simulink model "Demo_DSRC_DNPW_cs"  (Simulink 7.6)
settings: Solver=ode5  SolverMode=SingleTasking  StartTime=0.0  StopTime=5  FixedStep=1/20  RelTol=1e-3
PreLoadFcn:
  | check_NUTS_defined;
  | 
  | assignin('base',['model_closed_' bdroot],false);
InitFcn:
  | PreScanExperimentInitFcn(bdroot)
StopFcn:
  | PreScanExperimentStopFcn(bdroot)
undefined symbols (not defined in the file): DiscIntNeverNeededParam, spare_1, spare_10, spare_11, spare_12, spare_13, spare_14, spare_15, spare_16, spare_17, spare_18, spare_19, spare_2, spare_3, spare_4, spare_5, spare_6, spare_7, spare_8, spare_9
libraries: PreScanSimulinkLibrary x29, PreScanUsefulBlocks x11, simulink x9, simulink_extras x2
(part 5 of 6)

== system Demo_DSRC_DNPW_cs/STATE_Nissan_Cabstar_1/velRPY ==
  Y : Inport
  Assignment : Assignment  IndexMode=Zero-based  SampleTime=TimeStep  IndexOptions=Starting index (dialog)  Indices=PortIndex  OutputSizes=[1 1]
  Data Store Read : DataStoreRead  DataStoreName=SimCoreActuators  SampleTime=TimeStep
  Data Store Write : DataStoreWrite  DataStoreName=SimCoreActuators
  wires:
  Assignment/1 -> Data Store Write/1
  Data Store Read/1 -> Assignment/1
  Y/1 -> Assignment/2

== system Demo_DSRC_DNPW_cs/STATE_Toyota_Yaris_1/Acceleration ==
  Y : Inport
  Assignment : Assignment  IndexMode=Zero-based  SampleTime=TimeStep  IndexOptions=Starting index (dialog)  Indices=PortIndex  OutputSizes=[1 1]
  Data Store Read : DataStoreRead  DataStoreName=SimCoreActuators  SampleTime=TimeStep
  Data Store Write : DataStoreWrite  DataStoreName=SimCoreActuators
  wires:
  Assignment/1 -> Data Store Write/1
  Data Store Read/1 -> Assignment/1
  Y/1 -> Assignment/2

== system Demo_DSRC_DNPW_cs/STATE_Toyota_Yaris_1/Position ==
  Y : Inport
  Assignment : Assignment  IndexMode=Zero-based  SampleTime=TimeStep  IndexOptions=Starting index (dialog)  Indices=PortIndex  OutputSizes=[1 1]
  Data Store Read : DataStoreRead  DataStoreName=SimCoreActuators  SampleTime=TimeStep
  Data Store Write : DataStoreWrite  DataStoreName=SimCoreActuators
  wires:
  Y/1 -> Assignment/2
  Data Store Read/1 -> Assignment/1
  Assignment/1 -> Data Store Write/1

== system Demo_DSRC_DNPW_cs/STATE_Toyota_Yaris_1/RPY ==
  Y : Inport
  Assignment : Assignment  IndexMode=Zero-based  SampleTime=TimeStep  IndexOptions=Starting index (dialog)  Indices=PortIndex  OutputSizes=[1 1]
  Data Store Read : DataStoreRead  DataStoreName=SimCoreActuators  SampleTime=TimeStep
  Data Store Write : DataStoreWrite  DataStoreName=SimCoreActuators
  wires:
  Assignment/1 -> Data Store Write/1
  Data Store Read/1 -> Assignment/1
  Y/1 -> Assignment/2

== system Demo_DSRC_DNPW_cs/STATE_Toyota_Yaris_1/Velocity ==
  Y : Inport
  Assignment : Assignment  IndexMode=Zero-based  SampleTime=TimeStep  IndexOptions=Starting index (dialog)  Indices=PortIndex  OutputSizes=[1 1]
  Data Store Read : DataStoreRead  DataStoreName=SimCoreActuators  SampleTime=TimeStep
  Data Store Write : DataStoreWrite  DataStoreName=SimCoreActuators
  wires:
  Assignment/1 -> Data Store Write/1
  Data Store Read/1 -> Assignment/1
  Y/1 -> Assignment/2

== system Demo_DSRC_DNPW_cs/STATE_Toyota_Yaris_1/velRPY ==
  Y : Inport
  Assignment : Assignment  IndexMode=Zero-based  SampleTime=TimeStep  IndexOptions=Starting index (dialog)  Indices=PortIndex  OutputSizes=[1 1]
  Data Store Read : DataStoreRead  DataStoreName=SimCoreActuators  SampleTime=TimeStep
  Data Store Write : DataStoreWrite  DataStoreName=SimCoreActuators
  wires:
  Assignment/1 -> Data Store Write/1
  Data Store Read/1 -> Assignment/1
  Y/1 -> Assignment/2

== system Demo_DSRC_DNPW_cs/Toyota_Yaris_1/DSRC Transmitter ==
  Data : Inport
  Enable : EnablePort  PropagateVarSize=During execution
  DSRC_T_BusAssignment : BusAssignment  Tag=BusDSRCT  AssignedSignals=spare_1,spare_2,spare_3,spare_4,spare_5,spare_6,spare_7,spare_8,spare_9,spare_10,spare_11,spare_12,spare_13,spare_14,spare_15,spare_16,spare_17,spare_18,spare_19
  DSRC_T_Mux : Subsystem  Tag=MuxDSRCT
      settings: DeleteFcn=PreScanBlockDeleteFcn;
      mask Type: PreScan Mux Block:
      mask Display:
      | port_label('input', 1, 'Warning signal ID')
      | port_label('input', 2, 'Maneuvre ID')
      | port_label('input', 3, 'Vehicle Type')
      | port_label('input', 4, 'Braking Capacity')
      | port_label('input', 5, 'Vehicle Size')
      | port_label('input', 6, 'spare')
  Demux : Demux  Outputs=19
  Ground_{4..8} (5 alike) : Ground
  DSRC_T : Outport  Tag=AntennaTOutport
  wires:
  Demux/19 -> DSRC_T_BusAssignment/20  "Vehicle Height"
  Demux/18 -> DSRC_T_BusAssignment/19  "Vehicle Width"
  Demux/17 -> DSRC_T_BusAssignment/18  "Brakes"
  Demux/16 -> DSRC_T_BusAssignment/17  "Yaw rate"
  Demux/15 -> DSRC_T_BusAssignment/16  "Veritical Acc"
  Demux/14 -> DSRC_T_BusAssignment/15  "Lateral Acc"
  Demux/13 -> DSRC_T_BusAssignment/14  "Longitudinal Acc"
  Demux/12 -> DSRC_T_BusAssignment/13  "Angle"
  Demux/11 -> DSRC_T_BusAssignment/12  "Heading"
  Demux/10 -> DSRC_T_BusAssignment/11  "Speed"
  Demux/9 -> DSRC_T_BusAssignment/10  "Transmission State"
  Demux/8 -> DSRC_T_BusAssignment/9  "Accuracy"
  Demux/7 -> DSRC_T_BusAssignment/8  "Elevation"
  Demux/6 -> DSRC_T_BusAssignment/7  "Longitudinal"
  Demux/5 -> DSRC_T_BusAssignment/6  "Lateral"
  Ground_8/1 -> DSRC_T_Mux/5(vehicle_size)  "l50"
  Ground_7/1 -> DSRC_T_Mux/4(brakingcapacity)  "l49"
  Ground_6/1 -> DSRC_T_Mux/3(vehicle_type)  "l48"
  Ground_5/1 -> DSRC_T_Mux/2(maneuvre_id)  "l47"
  Ground_4/1 -> DSRC_T_Mux/1(warning_signal_id)  "l46"
  DSRC_T_Mux/1(Out1) -> DSRC_T/1  "l60"
  DSRC_T_BusAssignment/1 -> DSRC_T_Mux/6(spare)  "l58"
  Demux/4 -> DSRC_T_BusAssignment/5  "SecMark"
  Demux/3 -> DSRC_T_BusAssignment/4  "TempId"
  Demux/2 -> DSRC_T_BusAssignment/3  "MsgCount"
  Demux/1 -> DSRC_T_BusAssignment/2  "MsgId"
  Data/1 -> Demux/1
  DSRC_T_Mux/2(Out2) -> DSRC_T_BusAssignment/1  "L29"

== system Demo_DSRC_DNPW_cs/Toyota_Yaris_1/J2735 Encoder Basic Safety Message ==
  Msg : Inport
  Enable : EnablePort  PropagateVarSize=During execution
  Constant : Constant
  Demux : Demux  Outputs=19
  Embedded MATLAB Function : Stateflow chart  TreatAsAtomicUnit=on
  f() : Outport  InitialOutput=[1]
  Data : Outport  Port=2
  wires:
  Embedded MATLAB Function/1(y) -> Data/1
  Demux/19 -> Embedded MATLAB Function/19(u19)
  Demux/18 -> Embedded MATLAB Function/18(u18)
  Demux/17 -> Embedded MATLAB Function/17(u17)
  Demux/16 -> Embedded MATLAB Function/16(u16)
  Demux/15 -> Embedded MATLAB Function/15(u15)
  Demux/14 -> Embedded MATLAB Function/14(u14)
  Demux/13 -> Embedded MATLAB Function/13(u13)
  Demux/12 -> Embedded MATLAB Function/12(u12)
  Demux/11 -> Embedded MATLAB Function/11(u11)
  Demux/10 -> Embedded MATLAB Function/10(u10)
  Demux/9 -> Embedded MATLAB Function/9(u9)
  Demux/8 -> Embedded MATLAB Function/8(u8)
  Demux/7 -> Embedded MATLAB Function/7(u7)
  Demux/6 -> Embedded MATLAB Function/6(u6)
  Demux/5 -> Embedded MATLAB Function/5(u5)
  Demux/4 -> Embedded MATLAB Function/4(u4)
  Demux/3 -> Embedded MATLAB Function/3(u3)
  Demux/2 -> Embedded MATLAB Function/2(u2)
  Demux/1 -> Embedded MATLAB Function/1(u1)
  Constant/1 -> f()/1  "Enabled"
  Msg/1 -> Demux/1

== system Demo_DSRC_DNPW_cs/Toyota_Yaris_1/SELF_Demux ==
  SELF : Inport
  Demux1 : Demux  Outputs=3
  Demux2 : Demux  Outputs=3
  Demux3 : Demux  Outputs=[3 3 1 1]
  Demux4 : Demux  Outputs=3
  Gain : Gain  Gain=180/pi
  Gain1 : Gain  Gain=180/pi
  Selector : Selector  InputPortWidth=3  IndexOptions=Index vector (dialog)  Indices=[3]  OutputSizes=1
  compas converter : Subsystem
  xyz2GPS : PreScanUsefulBlocks/xyz2GPS  CoordinateCount=1  GPS_base=[0.000000 0.000000 0.000]
  x [m] : Outport
  y [m] : Outport  Port=2
  z [m] : Outport  Port=3
  rotx [deg] : Outport  Port=4
  roty [deg] : Outport  Port=5
  rotz [deg] : Outport  Port=6
  GPS lat [deg] : Outport  Port=7
  GPS long [deg] : Outport  Port=8
  GPS alt [m] : Outport  Port=9
  velocity [m/s] : Outport  Port=10
  heading [deg] : Outport  Port=11
  yaw rate [deg/s] : Outport  Port=12
  wires:
  Demux3/4 -> Gain1/1
  Gain1/1 -> yaw rate [deg/s]/1
  Demux3/3 -> velocity [m/s]/1
  compas converter/1(heading [deg]) -> heading [deg]/1
  xyz2GPS/1 -> Demux4/1
  Demux4/3 -> GPS alt [m]/1
  Demux4/2 -> GPS long [deg]/1
  Demux4/1 -> GPS lat [deg]/1
  Demux3/2 -> Gain/1, Selector/1
  Demux3/1 -> xyz2GPS/1, Demux1/1
  SELF/1 -> Demux3/1
  Demux2/3 -> rotz [deg]/1
  Demux2/2 -> roty [deg]/1
  Demux2/1 -> rotx [deg]/1
  Demux1/3 -> z [m]/1
  Demux1/2 -> y [m]/1
  Demux1/1 -> x [m]/1
  Gain/1 -> Demux2/1
  Selector/1 -> compas converter/1(rotz [rad])

== system Demo_DSRC_DNPW_cs/Toyota_Yaris_1/Trajectories ==
  Traj2State1 : Subsystem  Tag=Traj2State
      settings: DeleteFcn=PreScanBlockDeleteFcn;
      mask Type: PreScan Demux Block:
  Trajectory_1 : Subsystem  Tag=Trajectory  mask(PreScan Source Block: Trajectory){FileName='Trajectory_1_Synced.mat', TimeStep=1/20}
      mask prompts: TimeStep "Time Step [s]"
      mask help:
      | The Trajectory block contains the trajectories defined in the PreScan Experiment Editor. The output of the trajectory block is the (vehicle) State.
      |
      | For more information, please click Help.
      mask init: same as Demo_DSRC_DNPW_cs/BMW_X5_1/Trajectories/PathFollowerSva_2
      settings: DeleteFcn=PreScanBlockDeleteFcn;
      mask Help: eval('openHelp(312)')
      mask Display: fprintf(FileName)
  Trajectory_1_Offset : Constant  Tag=TrajectoryOffset  Value="[0  0  0  0  0  0]"
  State : Outport  Tag=TrajOutport
  wires:
  Trajectory_1/1(trajectory) -> Traj2State1/1(Traj Org)
  Trajectory_1_Offset/1 -> Traj2State1/2(Offset)
  Traj2State1/1(state) -> State/1

== system Demo_DSRC_DNPW_cs/Toyota_Yaris_1/VISUTextureColor_Mux ==
  RGB [-,-,-] : Inport
  TextureColor : Outport
  wires:
  RGB [-,-,-]/1 -> TextureColor/1

== system Demo_DSRC_DNPW_cs/VISUSteer_BMW_X5_1/conv_SteeringColumn ==
  angle [deg] : Inport
  Constant13 : Constant  Value=[0 1 0]
  Mux8 : Mux  Inputs=2
  deg2rad : Gain  Gain=pi/180
  QuaternionVisu [rad] : Outport
  wires:
  deg2rad/1 -> Mux8/2
  Constant13/1 -> Mux8/1
  Mux8/1 -> QuaternionVisu [rad]/1
  angle [deg]/1 -> deg2rad/1

== system Demo_DSRC_DNPW_cs/VISUSteer_BMW_X5_1/conv_SteeringWheel ==
  angle [deg] : Inport
  Constant13 : Constant  Value=[-1 0 0]
  Mux8 : Mux  Inputs=2
  deg2rad : Gain  Gain=pi/180
  QuaternionVisu [rad] : Outport
  wires:
  deg2rad/1 -> Mux8/2
  Constant13/1 -> Mux8/1
  Mux8/1 -> QuaternionVisu [rad]/1
  angle [deg]/1 -> deg2rad/1

== system Demo_DSRC_DNPW_cs/VISUSteer_BMW_X5_1/visu_SteeringColumn ==
  Y : Inport
  Assignment : Assignment  IndexMode=Zero-based  SampleTime=TimeStep  IndexOptions=Starting index (dialog)  Indices=PortIndex  OutputSizes=[1 1]
  Data Store Read : DataStoreRead  DataStoreName=SimCoreActuators  SampleTime=TimeStep
  Data Store Write : DataStoreWrite  DataStoreName=SimCoreActuators
  wires:
  Assignment/1 -> Data Store Write/1
  Data Store Read/1 -> Assignment/1
  Y/1 -> Assignment/2

== system Demo_DSRC_DNPW_cs/VISUSteer_BMW_X5_1/visu_SteeringWheel ==
  Y : Inport
  Assignment : Assignment  IndexMode=Zero-based  SampleTime=TimeStep  IndexOptions=Starting index (dialog)  Indices=PortIndex  OutputSizes=[1 1]
  Data Store Read : DataStoreRead  DataStoreName=SimCoreActuators  SampleTime=TimeStep
  Data Store Write : DataStoreWrite  DataStoreName=SimCoreActuators
  wires:
  Assignment/1 -> Data Store Write/1
  Data Store Read/1 -> Assignment/1
  Y/1 -> Assignment/2

== system Demo_DSRC_DNPW_cs/VISUTextureColor_Fiat_Bravo_1/visu_TextureColor ==
  Y : Inport
  Assignment : Assignment  IndexMode=Zero-based  SampleTime=TimeStep  IndexOptions=Starting index (dialog)  Indices=PortIndex  OutputSizes=[1 1]
  Data Store Read : DataStoreRead  DataStoreName=SimCoreActuators  SampleTime=TimeStep
  Data Store Write : DataStoreWrite  DataStoreName=SimCoreActuators
  wires:
  Assignment/1 -> Data Store Write/1
  Data Store Read/1 -> Assignment/1
  Y/1 -> Assignment/2

== system Demo_DSRC_DNPW_cs/VISUTextureColor_Toyota_Yaris_1/visu_TextureColor ==
  Y : Inport
  Assignment : Assignment  IndexMode=Zero-based  SampleTime=TimeStep  IndexOptions=Starting index (dialog)  Indices=PortIndex  OutputSizes=[1 1]
  Data Store Read : DataStoreRead  DataStoreName=SimCoreActuators  SampleTime=TimeStep
  Data Store Write : DataStoreWrite  DataStoreName=SimCoreActuators
  wires:
  Assignment/1 -> Data Store Write/1
  Data Store Read/1 -> Assignment/1
  Y/1 -> Assignment/2

== system Demo_DSRC_DNPW_cs/BMW_X5_1/DNPW/Forward Zone ==
  Range : Inport
  Theta : Inport  Port=2
  Abs : Abs
  Abs1 : Abs
  Logical Operator : Logic  Inputs=3  AllPortsSameDT=off  OutDataTypeStr=boolean
  Logical Operator1 : Logic  Operator=OR  Inputs=1  AllPortsSameDT=off  OutDataTypeStr=boolean
  Product : Product  RndMeth=Zero
  Relational Operator : RelationalOperator  Operator=<=  OutDataTypeStr=boolean
  Relational Operator1 : RelationalOperator  Operator=<=  OutDataTypeStr=boolean
  Relational Operator2 : RelationalOperator  Operator=<=  OutDataTypeStr=boolean
  Trigonometric Function : Trigonometry
  deg2rad : Gain  Gain=3.1415926/180
  Out1 : Outport
  wires:
  deg2rad/1 -> Trigonometric Function/1
  Range/1 -> Product/1, Relational Operator/1
  Trigonometric Function/1 -> Product/2
  Product/1 -> Abs/1
  Relational Operator/1 -> Logical Operator/1
  Relational Operator1/1 -> Logical Operator/2
  Logical Operator/1 -> Logical Operator1/1
  Theta/1 -> Abs1/1, deg2rad/1
  Relational Operator2/1 -> Logical Operator/3
  Logical Operator1/1 -> Out1/1
  [FZRange] -> Relational Operator/2
  Abs/1 -> Relational Operator1/1
  [FZHWidth] -> Relational Operator1/2
  Abs1/1 -> Relational Operator2/1
  [FZAngle] -> Relational Operator2/2

== system Demo_DSRC_DNPW_cs/BMW_X5_1/DNPW/Left Zone ==
  Range : Inport
  Theta : Inport  Port=2
  Abs : Abs
  Derivative : Derivative
  Logical Operator : Logic  Inputs=6  AllPortsSameDT=off  OutDataTypeStr=boolean
  Logical Operator1 : Logic  Operator=OR  Inputs=1  AllPortsSameDT=off  OutDataTypeStr=boolean
  Product : Product  RndMeth=Zero
  Relational Operator{,1,3,5} (4 alike) : RelationalOperator  Operator=<=  OutDataTypeStr=boolean
  Relational Operator2 : RelationalOperator  Operator=>  OutDataTypeStr=boolean
  Relational Operator4 : RelationalOperator  Operator=>  OutDataTypeStr=boolean
  Trigonometric Function : Trigonometry
  Unary Minus : UnaryMinus
  deg2rad : Gain  Gain=3.1415926/180
  Out1 : Outport
  wires:
  deg2rad/1 -> Trigonometric Function/1
  Range/1 -> Product/1, Derivative/1, Relational Operator/1
  Trigonometric Function/1 -> Product/2
  Product/1 -> Abs/1
  Abs/1 -> Relational Operator2/1, Relational Operator3/1
  Relational Operator/1 -> Logical Operator/1
  Logical Operator/1 -> Logical Operator1/1
  Theta/1 -> deg2rad/1, Relational Operator4/1, Relational Operator5/1
  Logical Operator1/1 -> Out1/1
  Relational Operator1/1 -> Logical Operator/2
  Relational Operator2/1 -> Logical Operator/3
  Relational Operator3/1 -> Logical Operator/4
  Relational Operator4/1 -> Logical Operator/5
  Relational Operator5/1 -> Logical Operator/6
  Derivative/1 -> Relational Operator1/1
  [SZRange] -> Relational Operator/2
  [SZRangedot] -> Unary Minus/1
  Unary Minus/1 -> Relational Operator1/2
  [SZHWidthMin] -> Relational Operator2/2
  [SZHWidthMax] -> Relational Operator3/2
  [SZAngleMin] -> Relational Operator4/2
  [SZAngleMax] -> Relational Operator5/2

== system Demo_DSRC_DNPW_cs/BMW_X5_1/DNPW/Right Zone ==
  Range : Inport
  Theta : Inport  Port=2
  Abs : Abs
  Derivative : Derivative
  Logical Operator : Logic  Inputs=6  AllPortsSameDT=off  OutDataTypeStr=boolean
  Logical Operator1 : Logic  Operator=OR  Inputs=1  AllPortsSameDT=off  OutDataTypeStr=boolean
  Product : Product  RndMeth=Zero
  Relational Operator : RelationalOperator  Operator=<=  OutDataTypeStr=boolean
  Relational Operator1 : RelationalOperator  Operator=<=  OutDataTypeStr=boolean
  Relational Operator2 : RelationalOperator  Operator=>  OutDataTypeStr=boolean
  Relational Operator3 : RelationalOperator  Operator=<=  OutDataTypeStr=boolean
  Relational Operator4 : RelationalOperator  Operator=<  OutDataTypeStr=boolean
  Relational Operator5 : RelationalOperator  OutDataTypeStr=boolean
  Trigonometric Function : Trigonometry
  Unary Minus : UnaryMinus
  Unary Minus1 : UnaryMinus
  Unary Minus2 : UnaryMinus
  deg2rad : Gain  Gain=3.1415926/180
  Out1 : Outport
  wires:
  deg2rad/1 -> Trigonometric Function/1
  Range/1 -> Product/1, Derivative/1, Relational Operator/1
  Trigonometric Function/1 -> Product/2
  Product/1 -> Abs/1
  Abs/1 -> Relational Operator2/1, Relational Operator3/1
  Relational Operator/1 -> Logical Operator/1
  Logical Operator/1 -> Logical Operator1/1
  Theta/1 -> deg2rad/1, Relational Operator4/1, Relational Operator5/1
  Logical Operator1/1 -> Out1/1
  Relational Operator1/1 -> Logical Operator/2
  Relational Operator2/1 -> Logical Operator/3
  Relational Operator3/1 -> Logical Operator/4
  Relational Operator4/1 -> Logical Operator/5
  Relational Operator5/1 -> Logical Operator/6
  Derivative/1 -> Relational Operator1/1
  [SZRange] -> Relational Operator/2
  [SZRangedot] -> Unary Minus/1
  Unary Minus/1 -> Relational Operator1/2
  [SZHWidthMin] -> Relational Operator2/2
  [SZHWidthMax] -> Relational Operator3/2
  [SZAngleMin] -> Unary Minus1/1
  [SZAngleMax] -> Unary Minus2/1
  Unary Minus1/1 -> Relational Operator4/2
  Unary Minus2/1 -> Relational Operator5/2

== system Demo_DSRC_DNPW_cs/BMW_X5_1/DNPW/Signal Delay ==
  In1 : Inport
  Compare To Zero : simulink/Logic and Bit Operations/Compare To Zero  SystemSampleTime=-1  relop=>  LogicOutDataTypeMode=uint8
  Constant : Constant  Value=10
  Constant1 : Constant
  Memory : Memory
  Sum : Sum  Inputs=|-+
  Switch : Switch  Criteria=u2 ~= 0
  Out1 : Outport
  wires:
  Constant/1 -> Switch/1
  Switch/1 -> Memory/1, Compare To Zero/1
  Memory/1 -> Sum/2
  Sum/1 -> Switch/3
  Constant1/1 -> Sum/1
  Compare To Zero/1 -> Out1/1
  In1/1 -> Switch/2

== system Demo_DSRC_DNPW_cs/BMW_X5_1/DNPW/Signal Delay1 ==
  In1 : Inport
  Compare To Zero : simulink/Logic and Bit Operations/Compare To Zero  SystemSampleTime=-1  relop=>  LogicOutDataTypeMode=uint8
  Constant : Constant  Value=10
  Constant1 : Constant
  Memory : Memory
  Sum : Sum  Inputs=|-+
  Switch : Switch  Criteria=u2 ~= 0
  Out1 : Outport
  wires:
  Constant/1 -> Switch/1
  Switch/1 -> Memory/1, Compare To Zero/1
  Memory/1 -> Sum/2
  Sum/1 -> Switch/3
  Constant1/1 -> Sum/1
  Compare To Zero/1 -> Out1/1
  In1/1 -> Switch/2

== system Demo_DSRC_DNPW_cs/BMW_X5_1/DNPW/Signal Delay2 ==
  In1 : Inport
  Compare To Zero : simulink/Logic and Bit Operations/Compare To Zero  SystemSampleTime=-1  relop=>  LogicOutDataTypeMode=uint8
  Constant : Constant  Value=10
  Constant1 : Constant
  Memory : Memory
  Sum : Sum  Inputs=|-+
  Switch : Switch  Criteria=u2 ~= 0
  Out1 : Outport
  wires:
  Constant/1 -> Switch/1
  Switch/1 -> Memory/1, Compare To Zero/1
  Memory/1 -> Sum/2
  Sum/1 -> Switch/3
  Constant1/1 -> Sum/1
  Compare To Zero/1 -> Out1/1
  In1/1 -> Switch/2

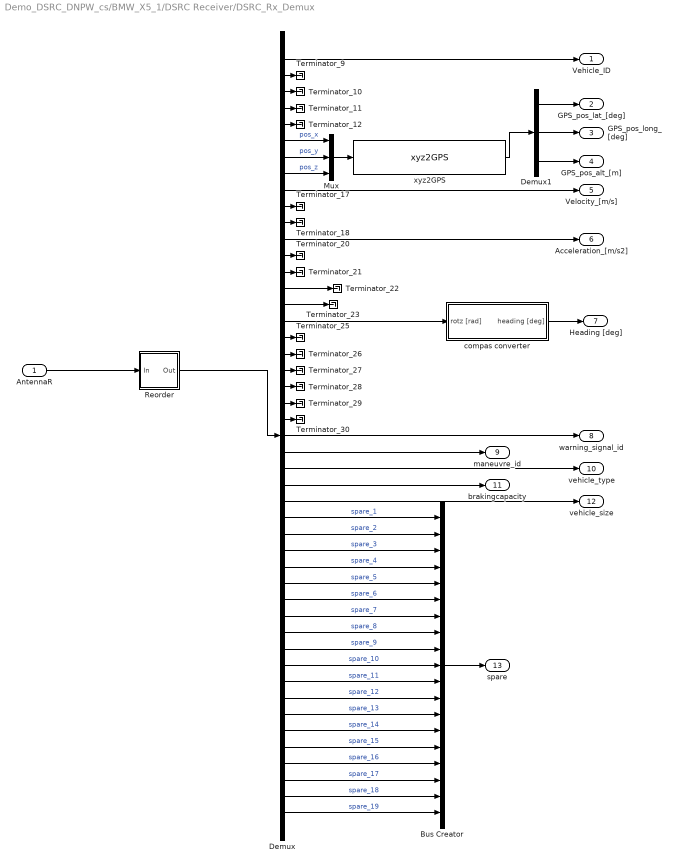
== system Demo_DSRC_DNPW_cs/BMW_X5_1/DSRC Receiver/DSRC_Rx_Demux ==
  AntennaR : Inport
  Bus Creator : BusCreator  Inputs=19
  Demux : Demux  Outputs=47
  Demux1 : Demux  Outputs=3
  Mux : Mux  Inputs=3
  Reorder : Subsystem  mask(Output reorder block){NrOfOutputs=47, NrOfObjects=3}
      mask prompts: NrOfOutputs "Number Of Outputs [-]"; NrOfObjects "Number Of Objects [-]"
      mask help: Change output order from object based to output type based
      mask init:
      | InputPortWidth=NrOfObjects*NrOfOutputs;
      | Input=1:InputPortWidth;
      | ReshapedInput=reshape(Input,NrOfOutputs,NrOfObjects);
      | TransposedReshapedInput=transpose(ReshapedInput);
      | Elements=reshape(TransposedReshapedInput,length(Input),1);
  Terminator_{9..12,17..18,20..23,25..30} (16 alike) : Terminator
  compas converter : Subsystem
  xyz2GPS : PreScanUsefulBlocks/xyz2GPS  CoordinateCount=3  GPS_base=[0.000000 0.000000 0.000]
  Vehicle_ID : Outport
  GPS_pos_lat_[deg] : Outport  Port=2
  GPS_pos_long_[deg] : Outport  Port=3
  GPS_pos_alt_[m] : Outport  Port=4
  Velocity_[m/s] : Outport  Port=5
  Acceleration_[m/s2] : Outport  Port=6
  Heading [deg] : Outport  Port=7
  warning_signal_id : Outport  Port=8
  maneuvre_id : Outport  Port=9
  vehicle_type : Outport  Port=10
  brakingcapacity : Outport  Port=11
  vehicle_size : Outport  Port=12
  spare : Outport  Port=13
  wires:
  Demux/47 -> Bus Creator/19  "spare_19"
  Demux/46 -> Bus Creator/18  "spare_18"
  Demux/45 -> Bus Creator/17  "spare_17"
  Demux/44 -> Bus Creator/16  "spare_16"
  Demux/43 -> Bus Creator/15  "spare_15"
  Demux/42 -> Bus Creator/14  "spare_14"
  Demux/41 -> Bus Creator/13  "spare_13"
  Demux/40 -> Bus Creator/12  "spare_12"
  Demux/39 -> Bus Creator/11  "spare_11"
  Demux/38 -> Bus Creator/10  "spare_10"
  Demux/37 -> Bus Creator/9  "spare_9"
  Demux/36 -> Bus Creator/8  "spare_8"
  Demux/35 -> Bus Creator/7  "spare_7"
  Demux/34 -> Bus Creator/6  "spare_6"
  Demux/33 -> Bus Creator/5  "spare_5"
  Demux/32 -> Bus Creator/4  "spare_4"
  Demux/31 -> Bus Creator/3  "spare_3"
  Demux/30 -> Bus Creator/2  "spare_2"
  Demux/29 -> Bus Creator/1  "spare_1"
  AntennaR/1 -> Reorder/1(In)
  Reorder/1(Out) -> Demux/1
  Mux/1 -> xyz2GPS/1
  Demux1/3 -> GPS_pos_alt_[m]/1
  Demux1/2 -> GPS_pos_long_[deg]/1
  Demux1/1 -> GPS_pos_lat_[deg]/1
  xyz2GPS/1 -> Demux1/1
  Demux/28 -> vehicle_size/1
  Demux/27 -> brakingcapacity/1
  Demux/26 -> vehicle_type/1
  Demux/25 -> maneuvre_id/1
  Demux/24 -> warning_signal_id/1
  Demux/9 -> Velocity_[m/s]/1
  Demux/23 -> Terminator_30/1
  Demux/22 -> Terminator_29/1
  Demux/21 -> Terminator_28/1
  Demux/20 -> Terminator_27/1
  Demux/19 -> Terminator_26/1
  Demux/18 -> Terminator_25/1
  Demux/17 -> compas converter/1(rotz [rad])
  Demux/16 -> Terminator_23/1
  Demux/15 -> Terminator_22/1
  Demux/14 -> Terminator_21/1
  Demux/13 -> Terminator_20/1
  Demux/12 -> Acceleration_[m/s2]/1
  Demux/11 -> Terminator_18/1
  Demux/10 -> Terminator_17/1
  Demux/8 -> Mux/3  "pos_z"
  Demux/7 -> Mux/2  "pos_y"
  Demux/6 -> Mux/1  "pos_x"
  Demux/5 -> Terminator_12/1
  Demux/4 -> Terminator_11/1
  Demux/3 -> Terminator_10/1
  Demux/2 -> Terminator_9/1
  Demux/1 -> Vehicle_ID/1
  compas converter/1(heading [deg]) -> Heading [deg]/1
  Bus Creator/1 -> spare/1

== system Demo_DSRC_DNPW_cs/BMW_X5_1/GPS to Relative Position/Angle reform 1  ==
  note: This block changes the heading range from [0 ... 360] to [-180 ...180]
      | Also, a heading of 0 means driving to the right side of the scenario (from top view)
  In1 : Inport
  Complex to Magnitude-Angle2 : ComplexToMagnitudeAngle  Output=Angle
  Magnitude-Angle to Complex1 : MagnitudeAngleToComplex  Input=Angle  ConstantPart=1
  Sum5 : Sum  Inputs=|++
  Unary Minus : UnaryMinus
  deg2rad : Gain  Gain=3.1415926/180
  degree : Constant  Value=-90
  rad2deg : Gain  Gain=180/3.1415926
  Out1 : Outport
  wires:
  degree/1 -> Sum5/2
  Sum5/1 -> Unary Minus/1
  Magnitude-Angle to Complex1/1 -> Complex to Magnitude-Angle2/1
  deg2rad/1 -> Magnitude-Angle to Complex1/1
  Complex to Magnitude-Angle2/1 -> rad2deg/1
  rad2deg/1 -> Out1/1
  In1/1 -> Sum5/1
  Unary Minus/1 -> deg2rad/1

== system Demo_DSRC_DNPW_cs/BMW_X5_1/GPS to Relative Position/Angle reform 2 ==
  note: This block changes the heading range from [0 ... 360] to [-180 ...180]
  In1 : Inport
  Complex to Magnitude-Angle2 : ComplexToMagnitudeAngle  Output=Angle
  Magnitude-Angle to Complex1 : MagnitudeAngleToComplex  Input=Angle  ConstantPart=1
  deg2rad : Gain  Gain=3.1415926/180
  rad2deg : Gain  Gain=180/3.1415926
  Out1 : Outport
  wires:
  Magnitude-Angle to Complex1/1 -> Complex to Magnitude-Angle2/1
  deg2rad/1 -> Magnitude-Angle to Complex1/1
  Complex to Magnitude-Angle2/1 -> rad2deg/1
  rad2deg/1 -> Out1/1
  In1/1 -> deg2rad/1

== system Demo_DSRC_DNPW_cs/BMW_X5_1/SELF_Demux/compas converter ==
  rotz [rad] : Inport
  cart2compas : Subsystem
  rad2deg : Gain  Gain=180/pi
  heading [deg] : Outport
  wires:
  cart2compas/1(heading [deg]) -> heading [deg]/1
  rotz [rad]/1 -> rad2deg/1
  rad2deg/1 -> cart2compas/1(Angle [deg])

== system Demo_DSRC_DNPW_cs/BMW_X5_1/Trajectories/ElapsedTrack1 ==
  Offset : Inport
  s : Inport  Port=2
  Mux : Mux  Inputs=3
  Mux1 : Mux  Inputs=3
  MuxState : Subsystem
  OffsetCor : Subsystem
  pitchAngle : Lookup  InputValues=s  Table=pitch  LookUpMeth=Interpolation-Use End Values
  rollAngle : Lookup  InputValues=s  Table=roll  LookUpMeth=Interpolation-Use End Values
  xpos : Lookup  InputValues=s  Table=x  LookUpMeth=Interpolation-Use End Values
  yawAngle : Lookup  InputValues=s  Table=yaw  LookUpMeth=Interpolation-Use End Values
  ypos : Lookup  InputValues=s  Table=y  LookUpMeth=Interpolation-Use End Values
  zpos : Lookup  InputValues=s  Table=z  LookUpMeth=Interpolation-Use End Values
  state : Outport
  wires:
  zpos/1 -> OffsetCor/3(z pos)
  rollAngle/1 -> OffsetCor/4(R angle)
  pitchAngle/1 -> OffsetCor/5(P angle)
  yawAngle/1 -> OffsetCor/6(Y angle)
  OffsetCor/6(Y angle_cor) -> Mux1/3
  OffsetCor/5(P angle_cor) -> Mux1/2
  OffsetCor/4(R angle_cor) -> Mux1/1
  OffsetCor/3(z pos_cor) -> Mux/3
  MuxState/1(State) -> state/1
  Mux/1 -> MuxState/1(xyzPos_[m])
  s/1 -> pitchAngle/1, yawAngle/1, rollAngle/1, zpos/1, ypos/1, xpos/1
  Offset/1 -> OffsetCor/7(Offset)
  xpos/1 -> OffsetCor/1(x pos)
  ypos/1 -> OffsetCor/2(y pos)
  OffsetCor/1(x pos_cor) -> Mux/1
  OffsetCor/2(y pos_cor) -> Mux/2
  Mux1/1 -> MuxState/2(RPYAngle_[rad])

== system Demo_DSRC_DNPW_cs/BMW_X5_1/Trajectories/PathFollowerSva_2 ==
  From Workspace : FromWorkspace  VariableName=trajectory  SampleTime=TimeStep  OutputAfterFinalValue=Holding final value
  From Workspace1 : FromWorkspace  VariableName=trajectory  SampleTime=TimeStep  OutputAfterFinalValue=Setting to zero
  Mux : Mux  Inputs=2
  Selector1 : Selector  InputPortWidth=24  IndexOptions=Index vector (dialog)  Indices=[7:18]  OutputSizes=1
  Selector9 : Selector  InputPortWidth=24  IndexOptions=Index vector (dialog)  Indices=[1:6]  OutputSizes=1
  trajectory : Outport
  wires:
  Selector1/1 -> Mux/2
  Selector9/1 -> Mux/1
  Mux/1 -> trajectory/1
  From Workspace1/1 -> Selector1/1
  From Workspace/1 -> Selector9/1

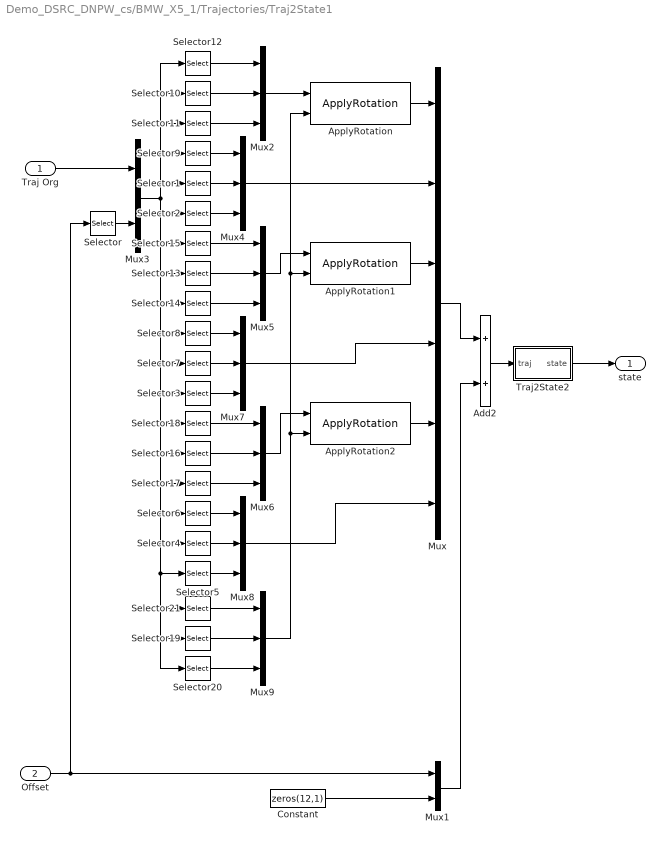
== system Demo_DSRC_DNPW_cs/BMW_X5_1/Trajectories/Traj2State1 ==
  Traj Org : Inport
  Offset : Inport  Port=2
  Add2 : Sum
  ApplyRotation : PreScanSimulinkLibrary/ApplyRotation  SystemSampleTime=-1
  ApplyRotation1 : PreScanSimulinkLibrary/ApplyRotation  SystemSampleTime=-1
  ApplyRotation2 : PreScanSimulinkLibrary/ApplyRotation  SystemSampleTime=-1
  Constant : Constant  Value=zeros(12,1)
  Mux : Mux  Inputs=6
  Mux1 : Mux  Inputs=2
  Mux{2,4..9} (7 alike) : Mux  Inputs=3
  Mux3 : Mux  Inputs=2
  Selector : Selector  InputPortWidth=6  IndexOptions=Index vector (dialog)  Indices=[4 5 6]  OutputSizes=1
  Selector1 : Selector  InputPortWidth=21  IndexOptions=Index vector (dialog)  Indices=[5]  OutputSizes=1
  Selector10 : Selector  InputPortWidth=21  IndexOptions=Index vector (dialog)  Indices=[2]  OutputSizes=1
  Selector11 : Selector  InputPortWidth=21  IndexOptions=Index vector (dialog)  Indices=[3]  OutputSizes=1
  Selector12 : Selector  InputPortWidth=21  IndexOptions=Index vector (dialog)  Indices=[1]  OutputSizes=1
  Selector13 : Selector  InputPortWidth=21  IndexOptions=Index vector (dialog)  Indices=[8]  OutputSizes=1
  Selector14 : Selector  InputPortWidth=21  IndexOptions=Index vector (dialog)  Indices=[9]  OutputSizes=1
  Selector15 : Selector  InputPortWidth=21  IndexOptions=Index vector (dialog)  Indices=[7]  OutputSizes=1
  Selector16 : Selector  InputPortWidth=21  IndexOptions=Index vector (dialog)  Indices=[14]  OutputSizes=1
  Selector17 : Selector  InputPortWidth=21  IndexOptions=Index vector (dialog)  Indices=[15]  OutputSizes=1
  Selector18 : Selector  InputPortWidth=21  IndexOptions=Index vector (dialog)  Indices=[13]  OutputSizes=1
  Selector19 : Selector  InputPortWidth=21  IndexOptions=Index vector (dialog)  Indices=[20]  OutputSizes=1
  Selector2 : Selector  InputPortWidth=21  IndexOptions=Index vector (dialog)  Indices=[6]  OutputSizes=1
  Selector20 : Selector  InputPortWidth=21  IndexOptions=Index vector (dialog)  Indices=[21]  OutputSizes=1
  Selector21 : Selector  InputPortWidth=21  IndexOptions=Index vector (dialog)  Indices=[19]  OutputSizes=1
  Selector3 : Selector  InputPortWidth=21  IndexOptions=Index vector (dialog)  Indices=[12]  OutputSizes=1
  Selector4 : Selector  InputPortWidth=21  IndexOptions=Index vector (dialog)  Indices=[17]  OutputSizes=1
  Selector5 : Selector  InputPortWidth=21  IndexOptions=Index vector (dialog)  Indices=[18]  OutputSizes=1
  Selector6 : Selector  InputPortWidth=21  IndexOptions=Index vector (dialog)  Indices=[16]  OutputSizes=1
  Selector7 : Selector  InputPortWidth=21  IndexOptions=Index vector (dialog)  Indices=[11]  OutputSizes=1
  Selector8 : Selector  InputPortWidth=21  IndexOptions=Index vector (dialog)  Indices=[10]  OutputSizes=1
  Selector9 : Selector  InputPortWidth=21  IndexOptions=Index vector (dialog)  Indices=[4]  OutputSizes=1
  Traj2State2 : Subsystem
  state : Outport
  wires:
  Mux9/1 -> ApplyRotation2/2, ApplyRotation1/2, ApplyRotation/2
  Selector20/1 -> Mux9/3
  Selector19/1 -> Mux9/2
  Selector21/1 -> Mux9/1
  Selector5/1 -> Mux8/3
  Selector4/1 -> Mux8/2
  Selector6/1 -> Mux8/1
  Mux8/1 -> Mux/6
  Mux6/1 -> ApplyRotation2/1
  Mux7/1 -> Mux/4
  ApplyRotation2/1 -> Mux/5
  Selector3/1 -> Mux7/3
  Selector7/1 -> Mux7/2
  Selector8/1 -> Mux7/1
  Mux4/1 -> Mux/2
  Mux5/1 -> ApplyRotation1/1
  ApplyRotation1/1 -> Mux/3
  Mux2/1 -> ApplyRotation/1
  ApplyRotation/1 -> Mux/1
  Selector2/1 -> Mux4/3
  Selector1/1 -> Mux4/2
  Selector9/1 -> Mux4/1
  Selector17/1 -> Mux6/3
  Selector16/1 -> Mux6/2
  Selector18/1 -> Mux6/1
  Selector14/1 -> Mux5/3
  Selector13/1 -> Mux5/2
  Selector15/1 -> Mux5/1
  Selector11/1 -> Mux2/3
  Selector10/1 -> Mux2/2
  Selector12/1 -> Mux2/1
  Mux3/1 -> Selector8/1, Selector7/1, Selector3/1, Selector18/1, Selector16/1, Selector17/1, Selector6/1, Selector20/1, Selector19/1, Selector21/1, Selector5/1, Selector4/1, Selector14/1, Selector13/1, Selector15/1, Selector2/1, Selector1/1, Selector9/1, Selector12/1, Selector10/1, Selector11/1
  Mux1/1 -> Add2/2
  Constant/1 -> Mux1/2
  Add2/1 -> Traj2State2/1(traj)
  Selector/1 -> Mux3/2
  Traj Org/1 -> Mux3/1
  Offset/1 -> Mux1/1, Selector/1
  Mux/1 -> Add2/1
  Traj2State2/1(state) -> state/1

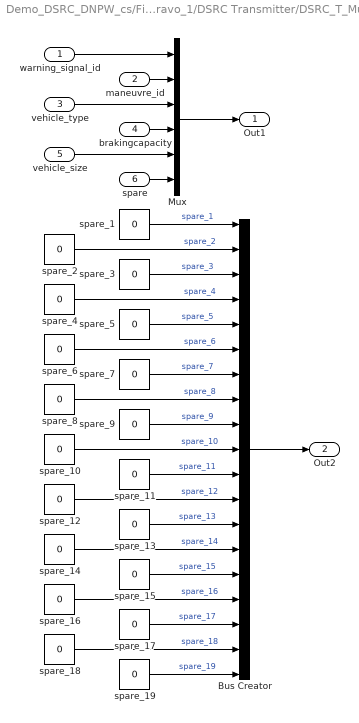
== system Demo_DSRC_DNPW_cs/Fiat_Bravo_1/DSRC Transmitter/DSRC_T_Mux ==
  warning_signal_id : Inport
  maneuvre_id : Inport  Port=2
  vehicle_type : Inport  Port=3
  brakingcapacity : Inport  Port=4
  vehicle_size : Inport  Port=5
  spare : Inport  Port=6
  Bus Creator : BusCreator  Inputs=19
  Mux : Mux  Inputs=6
  spare_{1..19} (19 alike) : Constant  Value=0
  Out1 : Outport
  Out2 : Outport  Port=2
  wires:
  spare_3/1 -> Bus Creator/3  "spare_3"
  spare_2/1 -> Bus Creator/2  "spare_2"
  spare_1/1 -> Bus Creator/1  "spare_1"
  spare_4/1 -> Bus Creator/4  "spare_4"
  spare/1 -> Mux/6
  Bus Creator/1 -> Out2/1
  Mux/1 -> Out1/1
  vehicle_size/1 -> Mux/5
  brakingcapacity/1 -> Mux/4
  vehicle_type/1 -> Mux/3
  maneuvre_id/1 -> Mux/2
  warning_signal_id/1 -> Mux/1
  spare_5/1 -> Bus Creator/5  "spare_5"
  spare_6/1 -> Bus Creator/6  "spare_6"
  spare_7/1 -> Bus Creator/7  "spare_7"
  spare_8/1 -> Bus Creator/8  "spare_8"
  spare_9/1 -> Bus Creator/9  "spare_9"
  spare_10/1 -> Bus Creator/10  "spare_10"
  spare_11/1 -> Bus Creator/11  "spare_11"
  spare_12/1 -> Bus Creator/12  "spare_12"
  spare_13/1 -> Bus Creator/13  "spare_13"
  spare_14/1 -> Bus Creator/14  "spare_14"
  spare_15/1 -> Bus Creator/15  "spare_15"
  spare_16/1 -> Bus Creator/16  "spare_16"
  spare_17/1 -> Bus Creator/17  "spare_17"
  spare_18/1 -> Bus Creator/18  "spare_18"
  spare_19/1 -> Bus Creator/19  "spare_19"

== system Demo_DSRC_DNPW_cs/Fiat_Bravo_1/SELF_Demux/compas converter ==
  rotz [rad] : Inport
  cart2compas : Subsystem
  rad2deg : Gain  Gain=180/pi
  heading [deg] : Outport
  wires:
  cart2compas/1(heading [deg]) -> heading [deg]/1
  rotz [rad]/1 -> rad2deg/1
  rad2deg/1 -> cart2compas/1(Angle [deg])

== system Demo_DSRC_DNPW_cs/Fiat_Bravo_1/Trajectories/PathFollowerSva_3 ==
  From Workspace : FromWorkspace  VariableName=trajectory  SampleTime=TimeStep  OutputAfterFinalValue=Holding final value
  From Workspace1 : FromWorkspace  VariableName=trajectory  SampleTime=TimeStep  OutputAfterFinalValue=Setting to zero
  Mux : Mux  Inputs=2
  Selector1 : Selector  InputPortWidth=24  IndexOptions=Index vector (dialog)  Indices=[7:18]  OutputSizes=1
  Selector9 : Selector  InputPortWidth=24  IndexOptions=Index vector (dialog)  Indices=[1:6]  OutputSizes=1
  trajectory : Outport
  wires:
  Selector1/1 -> Mux/2
  Selector9/1 -> Mux/1
  Mux/1 -> trajectory/1
  From Workspace1/1 -> Selector1/1
  From Workspace/1 -> Selector9/1

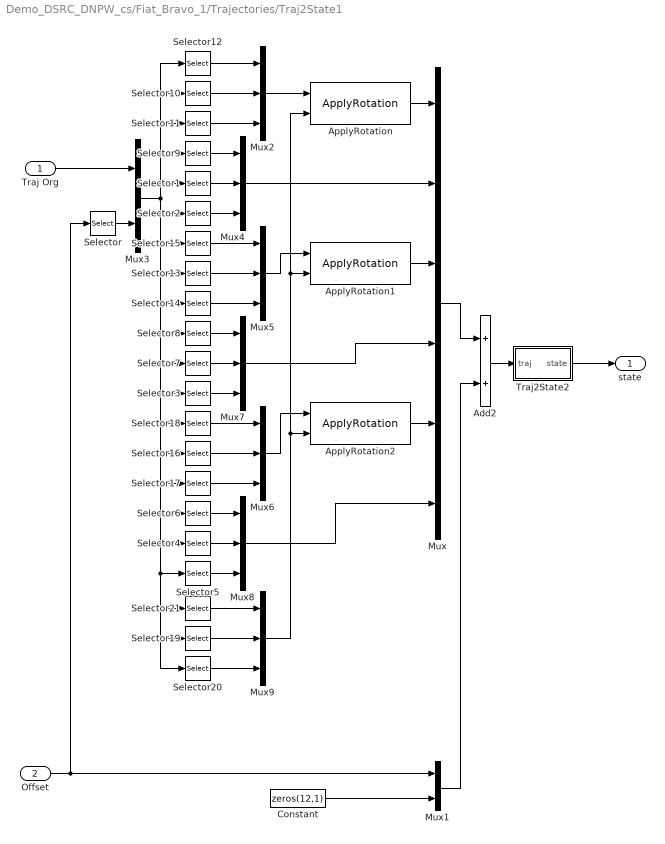
== system Demo_DSRC_DNPW_cs/Fiat_Bravo_1/Trajectories/Traj2State1 ==
  Traj Org : Inport
  Offset : Inport  Port=2
  Add2 : Sum
  ApplyRotation : PreScanSimulinkLibrary/ApplyRotation  SystemSampleTime=-1
  ApplyRotation1 : PreScanSimulinkLibrary/ApplyRotation  SystemSampleTime=-1
  ApplyRotation2 : PreScanSimulinkLibrary/ApplyRotation  SystemSampleTime=-1
  Constant : Constant  Value=zeros(12,1)
  Mux : Mux  Inputs=6
  Mux1 : Mux  Inputs=2
  Mux{2,4..9} (7 alike) : Mux  Inputs=3
  Mux3 : Mux  Inputs=2
  Selector : Selector  InputPortWidth=6  IndexOptions=Index vector (dialog)  Indices=[4 5 6]  OutputSizes=1
  Selector1 : Selector  InputPortWidth=21  IndexOptions=Index vector (dialog)  Indices=[5]  OutputSizes=1
  Selector10 : Selector  InputPortWidth=21  IndexOptions=Index vector (dialog)  Indices=[2]  OutputSizes=1
  Selector11 : Selector  InputPortWidth=21  IndexOptions=Index vector (dialog)  Indices=[3]  OutputSizes=1
  Selector12 : Selector  InputPortWidth=21  IndexOptions=Index vector (dialog)  Indices=[1]  OutputSizes=1
  Selector13 : Selector  InputPortWidth=21  IndexOptions=Index vector (dialog)  Indices=[8]  OutputSizes=1
  Selector14 : Selector  InputPortWidth=21  IndexOptions=Index vector (dialog)  Indices=[9]  OutputSizes=1
  Selector15 : Selector  InputPortWidth=21  IndexOptions=Index vector (dialog)  Indices=[7]  OutputSizes=1
  Selector16 : Selector  InputPortWidth=21  IndexOptions=Index vector (dialog)  Indices=[14]  OutputSizes=1
  Selector17 : Selector  InputPortWidth=21  IndexOptions=Index vector (dialog)  Indices=[15]  OutputSizes=1
  Selector18 : Selector  InputPortWidth=21  IndexOptions=Index vector (dialog)  Indices=[13]  OutputSizes=1
  Selector19 : Selector  InputPortWidth=21  IndexOptions=Index vector (dialog)  Indices=[20]  OutputSizes=1
  Selector2 : Selector  InputPortWidth=21  IndexOptions=Index vector (dialog)  Indices=[6]  OutputSizes=1
  Selector20 : Selector  InputPortWidth=21  IndexOptions=Index vector (dialog)  Indices=[21]  OutputSizes=1
  Selector21 : Selector  InputPortWidth=21  IndexOptions=Index vector (dialog)  Indices=[19]  OutputSizes=1
  Selector3 : Selector  InputPortWidth=21  IndexOptions=Index vector (dialog)  Indices=[12]  OutputSizes=1
  Selector4 : Selector  InputPortWidth=21  IndexOptions=Index vector (dialog)  Indices=[17]  OutputSizes=1
  Selector5 : Selector  InputPortWidth=21  IndexOptions=Index vector (dialog)  Indices=[18]  OutputSizes=1
  Selector6 : Selector  InputPortWidth=21  IndexOptions=Index vector (dialog)  Indices=[16]  OutputSizes=1
  Selector7 : Selector  InputPortWidth=21  IndexOptions=Index vector (dialog)  Indices=[11]  OutputSizes=1
  Selector8 : Selector  InputPortWidth=21  IndexOptions=Index vector (dialog)  Indices=[10]  OutputSizes=1
  Selector9 : Selector  InputPortWidth=21  IndexOptions=Index vector (dialog)  Indices=[4]  OutputSizes=1
  Traj2State2 : Subsystem
  state : Outport
  wires:
  Mux9/1 -> ApplyRotation2/2, ApplyRotation1/2, ApplyRotation/2
  Selector20/1 -> Mux9/3
  Selector19/1 -> Mux9/2
  Selector21/1 -> Mux9/1
  Selector5/1 -> Mux8/3
  Selector4/1 -> Mux8/2
  Selector6/1 -> Mux8/1
  Mux8/1 -> Mux/6
  Mux6/1 -> ApplyRotation2/1
  Mux7/1 -> Mux/4
  ApplyRotation2/1 -> Mux/5
  Selector3/1 -> Mux7/3
  Selector7/1 -> Mux7/2
  Selector8/1 -> Mux7/1
  Mux4/1 -> Mux/2
  Mux5/1 -> ApplyRotation1/1
  ApplyRotation1/1 -> Mux/3
  Mux2/1 -> ApplyRotation/1
  ApplyRotation/1 -> Mux/1
  Selector2/1 -> Mux4/3
  Selector1/1 -> Mux4/2
  Selector9/1 -> Mux4/1
  Selector17/1 -> Mux6/3
  Selector16/1 -> Mux6/2
  Selector18/1 -> Mux6/1
  Selector14/1 -> Mux5/3
  Selector13/1 -> Mux5/2
  Selector15/1 -> Mux5/1
  Selector11/1 -> Mux2/3
  Selector10/1 -> Mux2/2
  Selector12/1 -> Mux2/1
  Mux3/1 -> Selector8/1, Selector7/1, Selector3/1, Selector18/1, Selector16/1, Selector17/1, Selector6/1, Selector20/1, Selector19/1, Selector21/1, Selector5/1, Selector4/1, Selector14/1, Selector13/1, Selector15/1, Selector2/1, Selector1/1, Selector9/1, Selector12/1, Selector10/1, Selector11/1
  Mux1/1 -> Add2/2
  Constant/1 -> Mux1/2
  Add2/1 -> Traj2State2/1(traj)
  Selector/1 -> Mux3/2
  Traj Org/1 -> Mux3/1
  Offset/1 -> Mux1/1, Selector/1
  Mux/1 -> Add2/1
  Traj2State2/1(state) -> state/1

== system Demo_DSRC_DNPW_cs/HMI_Box_Left/Dynamics_Empty/MuxState ==
  note: mode: Dynamics
  note: mode: Positioning
  note: mode: Dynamics
      | VelVEHICLE
      | wrt VEH
  note: AnglesVEHICLE
      | wrtGLOB
  note: For state mode 'Dynamic' positions
      | are not taken into account, as they
      | are computed by integrating velocity.
      | Click annotation for Help.
  x [m] : Inport  SampleTime=TimeStep
  y [m] : Inport  Port=2  SampleTime=TimeStep
  z [m] : Inport  Port=3  SampleTime=TimeStep
  dx [m/s] : Inport  Port=4  SampleTime=TimeStep
  dy [m/s] : Inport  Port=5  SampleTime=TimeStep
  dz [m/s] : Inport  Port=6  SampleTime=TimeStep
  R [rad] : Inport  Port=7  SampleTime=TimeStep
  P [rad] : Inport  Port=8  SampleTime=TimeStep
  Y [rad] : Inport  Port=9  SampleTime=TimeStep
  Constant : Constant  DisableCoverage=on  Value=positioningmode
  Discrete-Time Integrator : DiscreteIntegrator  SampleTime=TimeStep  ICPrevOutput=DiscIntNeverNeededParam  ICPrevScaledInput=DiscIntNeverNeededParam
  Ground : Ground
  Ground1 : Ground
  Mux1 : Mux  Inputs=[3 3]
  Mux2 : Mux  Inputs=3
  Mux3 : Mux  Inputs=3
  Mux4 : Mux  Inputs=3
  Mux5 : Mux  Inputs=[3 3]
  Mux6 : Mux  Inputs=[6 3]
  Switch : Switch  Threshold=0.5
  Transformation_BODY2GLOBAL : PreScanSimulinkLibrary/Simple_Vehicle_Dynamics/Chassis/MuxDynState/Transformation_BODY2GLOBAL  SystemSampleTime=-1
  mux3 : Mux  Inputs=3
  state : Outport
  wires:
  Constant/1 -> Switch/2
  Mux6/1 -> state/1
  Mux4/1 -> Mux1/1
  Mux5/1 -> Switch/3
  Mux1/1 -> Switch/1
  Switch/1 -> Mux6/1  "PosVeh wrt  GLOB"
  P [rad]/1 -> Mux3/2
  R [rad]/1 -> Mux3/1
  dz [m/s]/1 -> Mux2/3
  dy [m/s]/1 -> Mux2/2
  dx [m/s]/1 -> Mux2/1
  z [m]/1 -> Mux4/3
  y [m]/1 -> Mux4/2
  x [m]/1 -> Mux4/1
  Ground1/1 -> mux3/2  "pitch"
  Y [rad]/1 -> mux3/3, Mux3/3  "yaw"
  Mux3/1 -> Mux6/2
  Transformation_BODY2GLOBAL/1 -> Discrete-Time Integrator/1, Mux5/2  "VelVEH wrt  GLOB"
  mux3/1 -> Transformation_BODY2GLOBAL/2
  Ground/1 -> mux3/1  "roll"
  Mux2/1 -> Mux1/2, Transformation_BODY2GLOBAL/1
  Discrete-Time Integrator/1 -> Mux5/1  "PosVEH wrt  GLOB"

== system Demo_DSRC_DNPW_cs/HMI_Box_Left/SELF_Demux/compas converter ==
  rotz [rad] : Inport
  cart2compas : Subsystem
  rad2deg : Gain  Gain=180/pi
  heading [deg] : Outport
  wires:
  cart2compas/1(heading [deg]) -> heading [deg]/1
  rotz [rad]/1 -> rad2deg/1
  rad2deg/1 -> cart2compas/1(Angle [deg])

== system Demo_DSRC_DNPW_cs/HMI_Box_Right/Dynamics_Empty/MuxState ==
  note: mode: Dynamics
  note: mode: Positioning
  note: mode: Dynamics
      | VelVEHICLE
      | wrt VEH
  note: AnglesVEHICLE
      | wrtGLOB
  note: For state mode 'Dynamic' positions
      | are not taken into account, as they
      | are computed by integrating velocity.
      | Click annotation for Help.
  x [m] : Inport  SampleTime=TimeStep
  y [m] : Inport  Port=2  SampleTime=TimeStep
  z [m] : Inport  Port=3  SampleTime=TimeStep
  dx [m/s] : Inport  Port=4  SampleTime=TimeStep
  dy [m/s] : Inport  Port=5  SampleTime=TimeStep
  dz [m/s] : Inport  Port=6  SampleTime=TimeStep
  R [rad] : Inport  Port=7  SampleTime=TimeStep
  P [rad] : Inport  Port=8  SampleTime=TimeStep
  Y [rad] : Inport  Port=9  SampleTime=TimeStep
  Constant : Constant  DisableCoverage=on  Value=positioningmode
  Discrete-Time Integrator : DiscreteIntegrator  SampleTime=TimeStep  ICPrevOutput=DiscIntNeverNeededParam  ICPrevScaledInput=DiscIntNeverNeededParam
  Ground : Ground
  Ground1 : Ground
  Mux1 : Mux  Inputs=[3 3]
  Mux2 : Mux  Inputs=3
  Mux3 : Mux  Inputs=3
  Mux4 : Mux  Inputs=3
  Mux5 : Mux  Inputs=[3 3]
  Mux6 : Mux  Inputs=[6 3]
  Switch : Switch  Threshold=0.5
  Transformation_BODY2GLOBAL : PreScanSimulinkLibrary/Simple_Vehicle_Dynamics/Chassis/MuxDynState/Transformation_BODY2GLOBAL  SystemSampleTime=-1
  mux3 : Mux  Inputs=3
  state : Outport
  wires:
  Constant/1 -> Switch/2
  Mux6/1 -> state/1
  Mux4/1 -> Mux1/1
  Mux5/1 -> Switch/3
  Mux1/1 -> Switch/1
  Switch/1 -> Mux6/1  "PosVeh wrt  GLOB"
  P [rad]/1 -> Mux3/2
  R [rad]/1 -> Mux3/1
  dz [m/s]/1 -> Mux2/3
  dy [m/s]/1 -> Mux2/2
  dx [m/s]/1 -> Mux2/1
  z [m]/1 -> Mux4/3
  y [m]/1 -> Mux4/2
  x [m]/1 -> Mux4/1
  Ground1/1 -> mux3/2  "pitch"
  Y [rad]/1 -> mux3/3, Mux3/3  "yaw"
  Mux3/1 -> Mux6/2
  Transformation_BODY2GLOBAL/1 -> Discrete-Time Integrator/1, Mux5/2  "VelVEH wrt  GLOB"
  mux3/1 -> Transformation_BODY2GLOBAL/2
  Ground/1 -> mux3/1  "roll"
  Mux2/1 -> Mux1/2, Transformation_BODY2GLOBAL/1
  Discrete-Time Integrator/1 -> Mux5/1  "PosVEH wrt  GLOB"

== system Demo_DSRC_DNPW_cs/HMI_Box_Right/SELF_Demux/compas converter ==
  rotz [rad] : Inport
  cart2compas : Subsystem
  rad2deg : Gain  Gain=180/pi
  heading [deg] : Outport
  wires:
  cart2compas/1(heading [deg]) -> heading [deg]/1
  rotz [rad]/1 -> rad2deg/1
  rad2deg/1 -> cart2compas/1(Angle [deg])

== system Demo_DSRC_DNPW_cs/HMI_Reminding_Left/Dynamics_Empty/MuxState ==
  note: mode: Dynamics
  note: mode: Positioning
  note: mode: Dynamics
      | VelVEHICLE
      | wrt VEH
  note: AnglesVEHICLE
      | wrtGLOB
  note: For state mode 'Dynamic' positions
      | are not taken into account, as they
      | are computed by integrating velocity.
      | Click annotation for Help.
  x [m] : Inport  SampleTime=TimeStep
  y [m] : Inport  Port=2  SampleTime=TimeStep
  z [m] : Inport  Port=3  SampleTime=TimeStep
  dx [m/s] : Inport  Port=4  SampleTime=TimeStep
  dy [m/s] : Inport  Port=5  SampleTime=TimeStep
  dz [m/s] : Inport  Port=6  SampleTime=TimeStep
  R [rad] : Inport  Port=7  SampleTime=TimeStep
  P [rad] : Inport  Port=8  SampleTime=TimeStep
  Y [rad] : Inport  Port=9  SampleTime=TimeStep
  Constant : Constant  DisableCoverage=on  Value=positioningmode
  Discrete-Time Integrator : DiscreteIntegrator  SampleTime=TimeStep  ICPrevOutput=DiscIntNeverNeededParam  ICPrevScaledInput=DiscIntNeverNeededParam
  Ground : Ground
  Ground1 : Ground
  Mux1 : Mux  Inputs=[3 3]
  Mux2 : Mux  Inputs=3
  Mux3 : Mux  Inputs=3
  Mux4 : Mux  Inputs=3
  Mux5 : Mux  Inputs=[3 3]
  Mux6 : Mux  Inputs=[6 3]
  Switch : Switch  Threshold=0.5
  Transformation_BODY2GLOBAL : PreScanSimulinkLibrary/Simple_Vehicle_Dynamics/Chassis/MuxDynState/Transformation_BODY2GLOBAL  SystemSampleTime=-1
  mux3 : Mux  Inputs=3
  state : Outport
  wires:
  Constant/1 -> Switch/2
  Mux6/1 -> state/1
  Mux4/1 -> Mux1/1
  Mux5/1 -> Switch/3
  Mux1/1 -> Switch/1
  Switch/1 -> Mux6/1  "PosVeh wrt  GLOB"
  P [rad]/1 -> Mux3/2
  R [rad]/1 -> Mux3/1
  dz [m/s]/1 -> Mux2/3
  dy [m/s]/1 -> Mux2/2
  dx [m/s]/1 -> Mux2/1
  z [m]/1 -> Mux4/3
  y [m]/1 -> Mux4/2
  x [m]/1 -> Mux4/1
  Ground1/1 -> mux3/2  "pitch"
  Y [rad]/1 -> mux3/3, Mux3/3  "yaw"
  Mux3/1 -> Mux6/2
  Transformation_BODY2GLOBAL/1 -> Discrete-Time Integrator/1, Mux5/2  "VelVEH wrt  GLOB"
  mux3/1 -> Transformation_BODY2GLOBAL/2
  Ground/1 -> mux3/1  "roll"
  Mux2/1 -> Mux1/2, Transformation_BODY2GLOBAL/1
  Discrete-Time Integrator/1 -> Mux5/1  "PosVEH wrt  GLOB"

== system Demo_DSRC_DNPW_cs/HMI_Reminding_Left/SELF_Demux/compas converter ==
  rotz [rad] : Inport
  cart2compas : Subsystem
  rad2deg : Gain  Gain=180/pi
  heading [deg] : Outport
  wires:
  cart2compas/1(heading [deg]) -> heading [deg]/1
  rotz [rad]/1 -> rad2deg/1
  rad2deg/1 -> cart2compas/1(Angle [deg])

== system Demo_DSRC_DNPW_cs/HMI_Reminding_Right/Dynamics_Empty/MuxState ==
  note: mode: Dynamics
  note: mode: Positioning
  note: mode: Dynamics
      | VelVEHICLE
      | wrt VEH
  note: AnglesVEHICLE
      | wrtGLOB
  note: For state mode 'Dynamic' positions
      | are not taken into account, as they
      | are computed by integrating velocity.
      | Click annotation for Help.
  x [m] : Inport  SampleTime=TimeStep
  y [m] : Inport  Port=2  SampleTime=TimeStep
  z [m] : Inport  Port=3  SampleTime=TimeStep
  dx [m/s] : Inport  Port=4  SampleTime=TimeStep
  dy [m/s] : Inport  Port=5  SampleTime=TimeStep
  dz [m/s] : Inport  Port=6  SampleTime=TimeStep
  R [rad] : Inport  Port=7  SampleTime=TimeStep
  P [rad] : Inport  Port=8  SampleTime=TimeStep
  Y [rad] : Inport  Port=9  SampleTime=TimeStep
  Constant : Constant  DisableCoverage=on  Value=positioningmode
  Discrete-Time Integrator : DiscreteIntegrator  SampleTime=TimeStep  ICPrevOutput=DiscIntNeverNeededParam  ICPrevScaledInput=DiscIntNeverNeededParam
  Ground : Ground
  Ground1 : Ground
  Mux1 : Mux  Inputs=[3 3]
  Mux2 : Mux  Inputs=3
  Mux3 : Mux  Inputs=3
  Mux4 : Mux  Inputs=3
  Mux5 : Mux  Inputs=[3 3]
  Mux6 : Mux  Inputs=[6 3]
  Switch : Switch  Threshold=0.5
  Transformation_BODY2GLOBAL : PreScanSimulinkLibrary/Simple_Vehicle_Dynamics/Chassis/MuxDynState/Transformation_BODY2GLOBAL  SystemSampleTime=-1
  mux3 : Mux  Inputs=3
  state : Outport
  wires:
  Constant/1 -> Switch/2
  Mux6/1 -> state/1
  Mux4/1 -> Mux1/1
  Mux5/1 -> Switch/3
  Mux1/1 -> Switch/1
  Switch/1 -> Mux6/1  "PosVeh wrt  GLOB"
  P [rad]/1 -> Mux3/2
  R [rad]/1 -> Mux3/1
  dz [m/s]/1 -> Mux2/3
  dy [m/s]/1 -> Mux2/2
  dx [m/s]/1 -> Mux2/1
  z [m]/1 -> Mux4/3
  y [m]/1 -> Mux4/2
  x [m]/1 -> Mux4/1
  Ground1/1 -> mux3/2  "pitch"
  Y [rad]/1 -> mux3/3, Mux3/3  "yaw"
  Mux3/1 -> Mux6/2
  Transformation_BODY2GLOBAL/1 -> Discrete-Time Integrator/1, Mux5/2  "VelVEH wrt  GLOB"
  mux3/1 -> Transformation_BODY2GLOBAL/2
  Ground/1 -> mux3/1  "roll"
  Mux2/1 -> Mux1/2, Transformation_BODY2GLOBAL/1
  Discrete-Time Integrator/1 -> Mux5/1  "PosVEH wrt  GLOB"

== system Demo_DSRC_DNPW_cs/HMI_Reminding_Right/SELF_Demux/compas converter ==
  rotz [rad] : Inport
  cart2compas : Subsystem
  rad2deg : Gain  Gain=180/pi
  heading [deg] : Outport
  wires:
  cart2compas/1(heading [deg]) -> heading [deg]/1
  rotz [rad]/1 -> rad2deg/1
  rad2deg/1 -> cart2compas/1(Angle [deg])

== system Demo_DSRC_DNPW_cs/HMI_Warning_Left/Dynamics_Empty/MuxState ==
  note: mode: Dynamics
  note: mode: Positioning
  note: mode: Dynamics
      | VelVEHICLE
      | wrt VEH
  note: AnglesVEHICLE
      | wrtGLOB
  note: For state mode 'Dynamic' positions
      | are not taken into account, as they
      | are computed by integrating velocity.
      | Click annotation for Help.
  x [m] : Inport  SampleTime=TimeStep
  y [m] : Inport  Port=2  SampleTime=TimeStep
  z [m] : Inport  Port=3  SampleTime=TimeStep
  dx [m/s] : Inport  Port=4  SampleTime=TimeStep
  dy [m/s] : Inport  Port=5  SampleTime=TimeStep
  dz [m/s] : Inport  Port=6  SampleTime=TimeStep
  R [rad] : Inport  Port=7  SampleTime=TimeStep
  P [rad] : Inport  Port=8  SampleTime=TimeStep
  Y [rad] : Inport  Port=9  SampleTime=TimeStep
  Constant : Constant  DisableCoverage=on  Value=positioningmode
  Discrete-Time Integrator : DiscreteIntegrator  SampleTime=TimeStep  ICPrevOutput=DiscIntNeverNeededParam  ICPrevScaledInput=DiscIntNeverNeededParam
  Ground : Ground
  Ground1 : Ground
  Mux1 : Mux  Inputs=[3 3]
  Mux2 : Mux  Inputs=3
  Mux3 : Mux  Inputs=3
  Mux4 : Mux  Inputs=3
  Mux5 : Mux  Inputs=[3 3]
  Mux6 : Mux  Inputs=[6 3]
  Switch : Switch  Threshold=0.5
  Transformation_BODY2GLOBAL : PreScanSimulinkLibrary/Simple_Vehicle_Dynamics/Chassis/MuxDynState/Transformation_BODY2GLOBAL  SystemSampleTime=-1
  mux3 : Mux  Inputs=3
  state : Outport
  wires:
  Constant/1 -> Switch/2
  Mux6/1 -> state/1
  Mux4/1 -> Mux1/1
  Mux5/1 -> Switch/3
  Mux1/1 -> Switch/1
  Switch/1 -> Mux6/1  "PosVeh wrt  GLOB"
  P [rad]/1 -> Mux3/2
  R [rad]/1 -> Mux3/1
  dz [m/s]/1 -> Mux2/3
  dy [m/s]/1 -> Mux2/2
  dx [m/s]/1 -> Mux2/1
  z [m]/1 -> Mux4/3
  y [m]/1 -> Mux4/2
  x [m]/1 -> Mux4/1
  Ground1/1 -> mux3/2  "pitch"
  Y [rad]/1 -> mux3/3, Mux3/3  "yaw"
  Mux3/1 -> Mux6/2
  Transformation_BODY2GLOBAL/1 -> Discrete-Time Integrator/1, Mux5/2  "VelVEH wrt  GLOB"
  mux3/1 -> Transformation_BODY2GLOBAL/2
  Ground/1 -> mux3/1  "roll"
  Mux2/1 -> Mux1/2, Transformation_BODY2GLOBAL/1
  Discrete-Time Integrator/1 -> Mux5/1  "PosVEH wrt  GLOB"

== system Demo_DSRC_DNPW_cs/HMI_Warning_Left/SELF_Demux/compas converter ==
  rotz [rad] : Inport
  cart2compas : Subsystem
  rad2deg : Gain  Gain=180/pi
  heading [deg] : Outport
  wires:
  cart2compas/1(heading [deg]) -> heading [deg]/1
  rotz [rad]/1 -> rad2deg/1
  rad2deg/1 -> cart2compas/1(Angle [deg])
